simulink model "Quadcopter"  (R2019a)
settings: Solver=VariableStepAuto  StartTime=0.0  StopTime=2000  MaxStep=1e-1  RelTol=1e-3
StopFcn:
  | hold on;
  | plot3(out.out_y1.data, out.out_x1.data, out.out_z1.data, 'r');
  | plot3(out.out_y2.data, out.out_x2.data, out.out_z2.data, 'g');
  | plot3(out.out_y3.data, out.out_x3.data, out.out_z3.data, 'b');
  | plot3([0;out.out_y.data(1:1000:end)], [0;out.out_x.data(1:1000:end)], [0;out.out_z.data(1:1000:end)], '.k');
  | view(3);
  | hold off;
values from neighbouring files (symbols this model uses):
  B_phi = 1    [Control.m]
  B_psi = 1    [Control.m]
  B_theta = 1    [Control.m]
  B_z = 5    [Control.m]
  r_x12 = 8    [Control.m]
  r_x32 = 4    [Control.m]
  r_y12 = 8    [Control.m]
  r_y32 = 4    [Control.m]
undefined symbols (not defined in the file or in its folder): As, Bs, Cpsi, Cs, Cx, Cy, Cz, Ds, x01, x02, x03, y01, y02, y03, z01, z02, z03
libraries: simulink x1
(part 2 of 3)

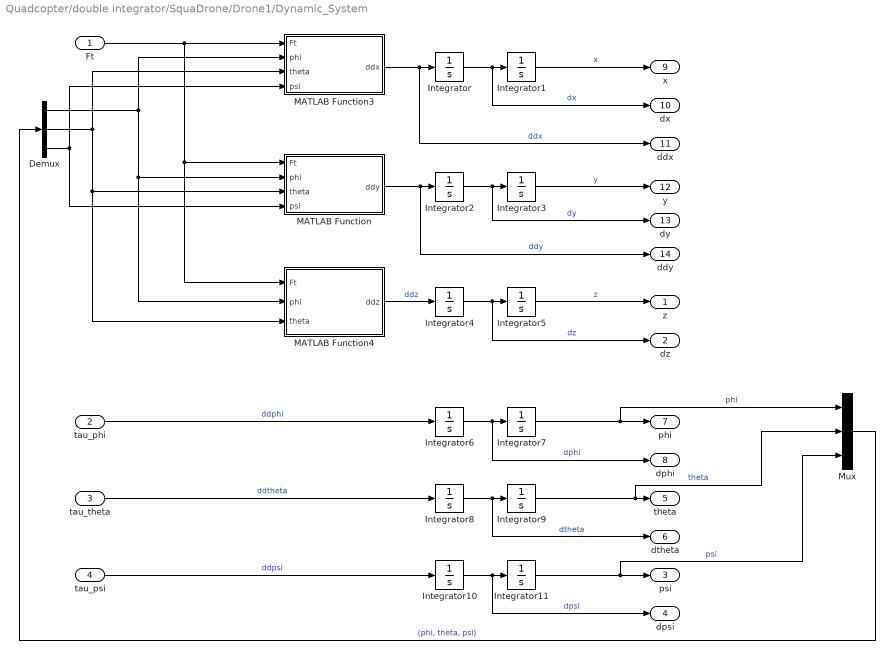
== system Quadcopter/double integrator/SquaDrone/Drone1/Dynamic_System ==
  Ft : Inport
  tau_phi : Inport  Port=2
  tau_theta : Inport  Port=3
  tau_psi : Inport  Port=4
  Demux : Demux  Outputs=3
  Integrator{,2,4,6..11} (9 alike) : Integrator
  Integrator1 : Integrator  InitialCondition=x01
  Integrator3 : Integrator  InitialCondition=y01
  Integrator5 : Integrator  InitialCondition=z01
  MATLAB Function : MATLAB Function  TreatAsAtomicUnit=on
  MATLAB Function3 : MATLAB Function  TreatAsAtomicUnit=on
  MATLAB Function4 : MATLAB Function  TreatAsAtomicUnit=on
  Mux : Mux  Inputs=3
  z : Outport
  dz : Outport  Port=2
  psi : Outport  Port=3
  dpsi : Outport  Port=4
  theta : Outport  Port=5
  dtheta : Outport  Port=6
  phi : Outport  Port=7
  dphi : Outport  Port=8
  x : Outport  Port=9
  dx : Outport  Port=10
  ddx : Outport  Port=11
  y : Outport  Port=12
  dy : Outport  Port=13
  ddy : Outport  Port=14
  wires:
  MATLAB Function3/1(ddx) -> ddx/1, Integrator/1  "ddx"
  Ft/1 -> MATLAB Function3/1(Ft), MATLAB Function4/1(Ft), MATLAB Function/1(Ft)
  Integrator/1 -> dx/1, Integrator1/1  "dx"
  Integrator1/1 -> x/1  "x"
  MATLAB Function/1(ddy) -> ddy/1, Integrator2/1  "ddy"
  Integrator2/1 -> dy/1, Integrator3/1  "dy"
  Integrator3/1 -> y/1  "y"
  MATLAB Function4/1(ddz) -> Integrator4/1  "ddz"
  Integrator4/1 -> dz/1, Integrator5/1  "dz"
  Integrator5/1 -> z/1  "z"
  tau_phi/1 -> Integrator6/1  "ddphi"
  Integrator6/1 -> dphi/1, Integrator7/1  "dphi"
  Integrator7/1 -> Mux/1, phi/1  "phi"
  Integrator9/1 -> Mux/2, theta/1  "theta"
  Integrator8/1 -> dtheta/1, Integrator9/1  "dtheta"
  tau_theta/1 -> Integrator8/1  "ddtheta"
  Integrator11/1 -> Mux/3, psi/1  "psi"
  Integrator10/1 -> dpsi/1, Integrator11/1  "dpsi"
  tau_psi/1 -> Integrator10/1  "ddpsi"
  Mux/1 -> Demux/1  "(phi, theta, psi)"
  Demux/1 -> MATLAB Function3/2(phi), MATLAB Function4/2(phi), MATLAB Function/2(phi)
  Demux/2 -> MATLAB Function3/3(theta), MATLAB Function4/3(theta), MATLAB Function/3(theta)
  Demux/3 -> MATLAB Function/4(psi), MATLAB Function3/4(psi)

== system Quadcopter/double integrator/SquaDrone/Drone2/Controller ==
  z : Inport
  dz : Inport  Port=2
  psi : Inport  Port=3
  dpsi : Inport  Port=4
  theta : Inport  Port=5
  dtheta : Inport  Port=6
  phi : Inport  Port=7
  dphi : Inport  Port=8
  zd : Inport  Port=9
  psid : Inport  Port=10
  thetad : Inport  Port=11
  dthetad : Inport  Port=12
  phid : Inport  Port=13
  dphid : Inport  Port=14
  Constant1 : Constant  Value=B_theta
  Constant14 : Constant  Value=B_z
  Constant20 : Constant  Value=B_psi
  Constant5 : Constant  Value=B_phi
  Gain{1,3,7..8} (4 alike) : Gain  Gain=2
  altitude : MATLAB Function  TreatAsAtomicUnit=on
  heading : MATLAB Function  TreatAsAtomicUnit=on
  lateral : MATLAB Function  TreatAsAtomicUnit=on
  longitudial : MATLAB Function  TreatAsAtomicUnit=on
  Ft : Outport
  tau_phi : Outport  Port=2
  tau_theta : Outport  Port=3
  tau_psi : Outport  Port=4
  wires:
  altitude/1(Ft) -> Ft/1
  longitudial/1(tau_phi) -> tau_phi/1
  lateral/1(tau_theta) -> tau_theta/1
  heading/1(tau_psi) -> tau_psi/1
  Gain7/1 -> altitude/7(M2)
  Constant14/1 -> Gain7/1, altitude/6(M1)
  Constant20/1 -> Gain8/1, heading/4(M1)
  Gain8/1 -> heading/5(M2)
  psid/1 -> heading/1(psid)
  psi/1 -> heading/2(psi)
  dpsi/1 -> heading/3(dpsi)
  theta/1 -> lateral/1(theta), altitude/4(theta)
  dtheta/1 -> lateral/2(dtheta)
  phi/1 -> longitudial/1(phi), altitude/3(phi)
  dphi/1 -> longitudial/2(dphi)
  zd/1 -> altitude/5(zd)
  z/1 -> altitude/1(z)
  dz/1 -> altitude/2(dz)
  Constant5/1 -> Gain3/1, longitudial/5(M1)
  Gain3/1 -> longitudial/6(M2)
  Constant1/1 -> Gain1/1, lateral/5(M1)
  Gain1/1 -> lateral/6(M2)
  thetad/1 -> lateral/3(thetad)
  dthetad/1 -> lateral/4(dthetad)
  phid/1 -> longitudial/3(phid)
  dphid/1 -> longitudial/4(dphid)

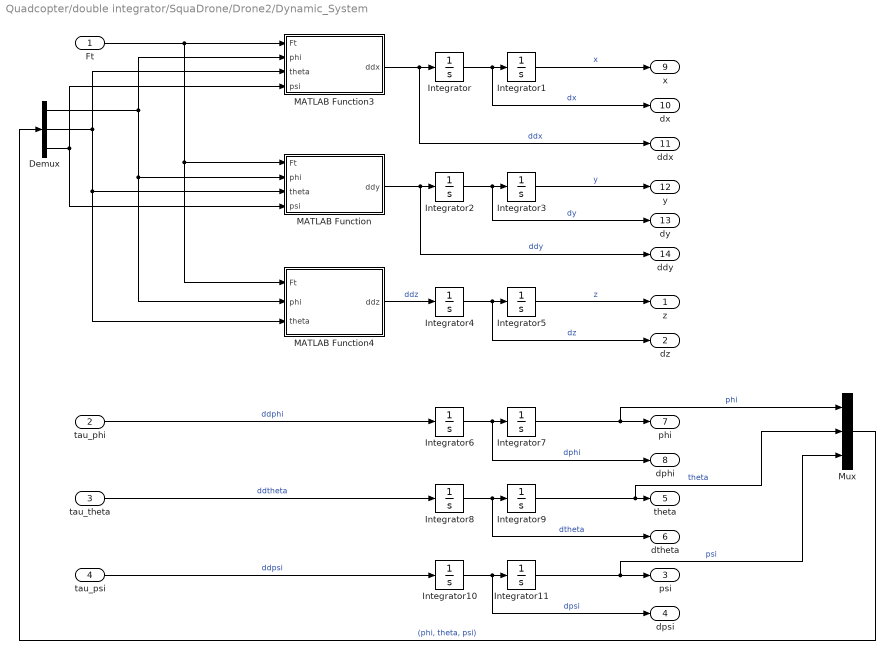
== system Quadcopter/double integrator/SquaDrone/Drone2/Dynamic_System ==
  Ft : Inport
  tau_phi : Inport  Port=2
  tau_theta : Inport  Port=3
  tau_psi : Inport  Port=4
  Demux : Demux  Outputs=3
  Integrator{,2,4,6..11} (9 alike) : Integrator
  Integrator1 : Integrator  InitialCondition=x02
  Integrator3 : Integrator  InitialCondition=y02
  Integrator5 : Integrator  InitialCondition=z02
  MATLAB Function : MATLAB Function  TreatAsAtomicUnit=on
  MATLAB Function3 : MATLAB Function  TreatAsAtomicUnit=on
  MATLAB Function4 : MATLAB Function  TreatAsAtomicUnit=on
  Mux : Mux  Inputs=3
  z : Outport
  dz : Outport  Port=2
  psi : Outport  Port=3
  dpsi : Outport  Port=4
  theta : Outport  Port=5
  dtheta : Outport  Port=6
  phi : Outport  Port=7
  dphi : Outport  Port=8
  x : Outport  Port=9
  dx : Outport  Port=10
  ddx : Outport  Port=11
  y : Outport  Port=12
  dy : Outport  Port=13
  ddy : Outport  Port=14
  wires:
  MATLAB Function3/1(ddx) -> ddx/1, Integrator/1  "ddx"
  Ft/1 -> MATLAB Function3/1(Ft), MATLAB Function4/1(Ft), MATLAB Function/1(Ft)
  Integrator/1 -> dx/1, Integrator1/1  "dx"
  Integrator1/1 -> x/1  "x"
  MATLAB Function/1(ddy) -> ddy/1, Integrator2/1  "ddy"
  Integrator2/1 -> dy/1, Integrator3/1  "dy"
  Integrator3/1 -> y/1  "y"
  MATLAB Function4/1(ddz) -> Integrator4/1  "ddz"
  Integrator4/1 -> dz/1, Integrator5/1  "dz"
  Integrator5/1 -> z/1  "z"
  tau_phi/1 -> Integrator6/1  "ddphi"
  Integrator6/1 -> dphi/1, Integrator7/1  "dphi"
  Integrator7/1 -> Mux/1, phi/1  "phi"
  Integrator9/1 -> Mux/2, theta/1  "theta"
  Integrator8/1 -> dtheta/1, Integrator9/1  "dtheta"
  tau_theta/1 -> Integrator8/1  "ddtheta"
  Integrator11/1 -> Mux/3, psi/1  "psi"
  Integrator10/1 -> dpsi/1, Integrator11/1  "dpsi"
  tau_psi/1 -> Integrator10/1  "ddpsi"
  Mux/1 -> Demux/1  "(phi, theta, psi)"
  Demux/1 -> MATLAB Function3/2(phi), MATLAB Function4/2(phi), MATLAB Function/2(phi)
  Demux/2 -> MATLAB Function3/3(theta), MATLAB Function4/3(theta), MATLAB Function/3(theta)
  Demux/3 -> MATLAB Function/4(psi), MATLAB Function3/4(psi)

== system Quadcopter/double integrator/SquaDrone/Drone3/Controller ==
  z : Inport
  dz : Inport  Port=2
  psi : Inport  Port=3
  dpsi : Inport  Port=4
  theta : Inport  Port=5
  dtheta : Inport  Port=6
  phi : Inport  Port=7
  dphi : Inport  Port=8
  zd : Inport  Port=9
  psid : Inport  Port=10
  thetad : Inport  Port=11
  dthetad : Inport  Port=12
  phid : Inport  Port=13
  dphid : Inport  Port=14
  Constant1 : Constant  Value=B_theta
  Constant14 : Constant  Value=B_z
  Constant20 : Constant  Value=B_psi
  Constant5 : Constant  Value=B_phi
  Gain{1,3,7..8} (4 alike) : Gain  Gain=2
  altitude : MATLAB Function  TreatAsAtomicUnit=on
  heading : MATLAB Function  TreatAsAtomicUnit=on
  lateral : MATLAB Function  TreatAsAtomicUnit=on
  longitudial : MATLAB Function  TreatAsAtomicUnit=on
  Ft : Outport
  tau_phi : Outport  Port=2
  tau_theta : Outport  Port=3
  tau_psi : Outport  Port=4
  wires:
  altitude/1(Ft) -> Ft/1
  longitudial/1(tau_phi) -> tau_phi/1
  lateral/1(tau_theta) -> tau_theta/1
  heading/1(tau_psi) -> tau_psi/1
  Gain7/1 -> altitude/7(M2)
  Constant14/1 -> Gain7/1, altitude/6(M1)
  Constant20/1 -> Gain8/1, heading/4(M1)
  Gain8/1 -> heading/5(M2)
  psid/1 -> heading/1(psid)
  psi/1 -> heading/2(psi)
  dpsi/1 -> heading/3(dpsi)
  theta/1 -> lateral/1(theta), altitude/4(theta)
  dtheta/1 -> lateral/2(dtheta)
  phi/1 -> longitudial/1(phi), altitude/3(phi)
  dphi/1 -> longitudial/2(dphi)
  zd/1 -> altitude/5(zd)
  z/1 -> altitude/1(z)
  dz/1 -> altitude/2(dz)
  Constant5/1 -> Gain3/1, longitudial/5(M1)
  Gain3/1 -> longitudial/6(M2)
  Constant1/1 -> Gain1/1, lateral/5(M1)
  Gain1/1 -> lateral/6(M2)
  thetad/1 -> lateral/3(thetad)
  dthetad/1 -> lateral/4(dthetad)
  phid/1 -> longitudial/3(phid)
  dphid/1 -> longitudial/4(dphid)

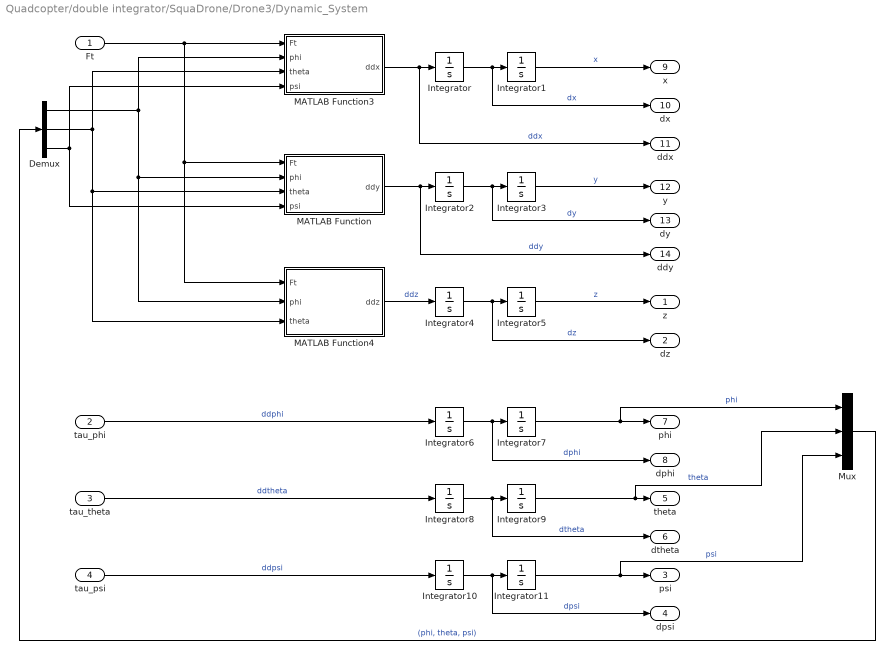
== system Quadcopter/double integrator/SquaDrone/Drone3/Dynamic_System ==
  Ft : Inport
  tau_phi : Inport  Port=2
  tau_theta : Inport  Port=3
  tau_psi : Inport  Port=4
  Demux : Demux  Outputs=3
  Integrator{,2,4,6..11} (9 alike) : Integrator
  Integrator1 : Integrator  InitialCondition=x03
  Integrator3 : Integrator  InitialCondition=y03
  Integrator5 : Integrator  InitialCondition=z03
  MATLAB Function : MATLAB Function  TreatAsAtomicUnit=on
  MATLAB Function3 : MATLAB Function  TreatAsAtomicUnit=on
  MATLAB Function4 : MATLAB Function  TreatAsAtomicUnit=on
  Mux : Mux  Inputs=3
  z : Outport
  dz : Outport  Port=2
  psi : Outport  Port=3
  dpsi : Outport  Port=4
  theta : Outport  Port=5
  dtheta : Outport  Port=6
  phi : Outport  Port=7
  dphi : Outport  Port=8
  x : Outport  Port=9
  dx : Outport  Port=10
  ddx : Outport  Port=11
  y : Outport  Port=12
  dy : Outport  Port=13
  ddy : Outport  Port=14
  wires:
  MATLAB Function3/1(ddx) -> ddx/1, Integrator/1  "ddx"
  Ft/1 -> MATLAB Function3/1(Ft), MATLAB Function4/1(Ft), MATLAB Function/1(Ft)
  Integrator/1 -> dx/1, Integrator1/1  "dx"
  Integrator1/1 -> x/1  "x"
  MATLAB Function/1(ddy) -> ddy/1, Integrator2/1  "ddy"
  Integrator2/1 -> dy/1, Integrator3/1  "dy"
  Integrator3/1 -> y/1  "y"
  MATLAB Function4/1(ddz) -> Integrator4/1  "ddz"
  Integrator4/1 -> dz/1, Integrator5/1  "dz"
  Integrator5/1 -> z/1  "z"
  tau_phi/1 -> Integrator6/1  "ddphi"
  Integrator6/1 -> dphi/1, Integrator7/1  "dphi"
  Integrator7/1 -> Mux/1, phi/1  "phi"
  Integrator9/1 -> Mux/2, theta/1  "theta"
  Integrator8/1 -> dtheta/1, Integrator9/1  "dtheta"
  tau_theta/1 -> Integrator8/1  "ddtheta"
  Integrator11/1 -> Mux/3, psi/1  "psi"
  Integrator10/1 -> dpsi/1, Integrator11/1  "dpsi"
  tau_psi/1 -> Integrator10/1  "ddpsi"
  Mux/1 -> Demux/1  "(phi, theta, psi)"
  Demux/1 -> MATLAB Function3/2(phi), MATLAB Function4/2(phi), MATLAB Function/2(phi)
  Demux/2 -> MATLAB Function3/3(theta), MATLAB Function4/3(theta), MATLAB Function/3(theta)
  Demux/3 -> MATLAB Function/4(psi), MATLAB Function3/4(psi)

== system Quadcopter/scheme - double integrator/SquaDrone/Drone1/Controller ==
  z : Inport
  dz : Inport  Port=2
  psi : Inport  Port=3
  dpsi : Inport  Port=4
  theta : Inport  Port=5
  dtheta : Inport  Port=6
  phi : Inport  Port=7
  dphi : Inport  Port=8
  zd : Inport  Port=9
  psid : Inport  Port=10
  thetad : Inport  Port=11
  dthetad : Inport  Port=12
  phid : Inport  Port=13
  dphid : Inport  Port=14
  Constant1 : Constant  Value=B_theta
  Constant14 : Constant  Value=B_z
  Constant20 : Constant  Value=B_psi
  Constant5 : Constant  Value=B_phi
  Gain{1,3,7..8} (4 alike) : Gain  Gain=2
  altitude : MATLAB Function  TreatAsAtomicUnit=on
  heading : MATLAB Function  TreatAsAtomicUnit=on
  lateral : MATLAB Function  TreatAsAtomicUnit=on
  longitudial : MATLAB Function  TreatAsAtomicUnit=on
  Ft : Outport
  tau_phi : Outport  Port=2
  tau_theta : Outport  Port=3
  tau_psi : Outport  Port=4
  wires:
  altitude/1(Ft) -> Ft/1
  longitudial/1(tau_phi) -> tau_phi/1
  lateral/1(tau_theta) -> tau_theta/1
  heading/1(tau_psi) -> tau_psi/1
  Gain7/1 -> altitude/7(M2)
  Constant14/1 -> Gain7/1, altitude/6(M1)
  Constant20/1 -> Gain8/1, heading/4(M1)
  Gain8/1 -> heading/5(M2)
  psid/1 -> heading/1(psid)
  psi/1 -> heading/2(psi)
  dpsi/1 -> heading/3(dpsi)
  theta/1 -> lateral/1(theta), altitude/4(theta)
  dtheta/1 -> lateral/2(dtheta)
  phi/1 -> longitudial/1(phi), altitude/3(phi)
  dphi/1 -> longitudial/2(dphi)
  zd/1 -> altitude/5(zd)
  z/1 -> altitude/1(z)
  dz/1 -> altitude/2(dz)
  Constant5/1 -> Gain3/1, longitudial/5(M1)
  Gain3/1 -> longitudial/6(M2)
  Constant1/1 -> Gain1/1, lateral/5(M1)
  Gain1/1 -> lateral/6(M2)
  thetad/1 -> lateral/3(thetad)
  dthetad/1 -> lateral/4(dthetad)
  phid/1 -> longitudial/3(phid)
  dphid/1 -> longitudial/4(dphid)

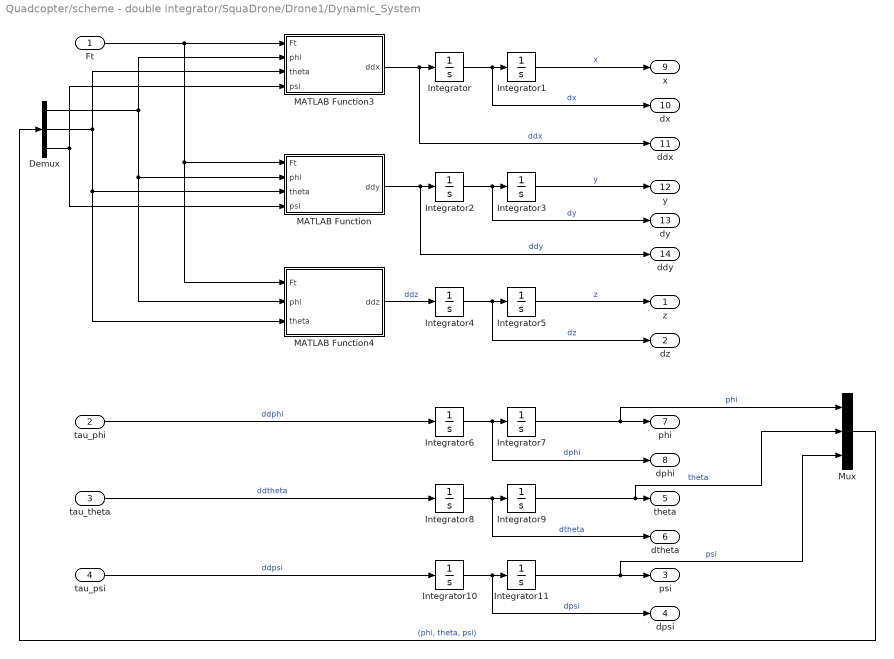
== system Quadcopter/scheme - double integrator/SquaDrone/Drone1/Dynamic_System ==
  Ft : Inport
  tau_phi : Inport  Port=2
  tau_theta : Inport  Port=3
  tau_psi : Inport  Port=4
  Demux : Demux  Outputs=3
  Integrator{,2,4,6..11} (9 alike) : Integrator
  Integrator1 : Integrator  InitialCondition=x01
  Integrator3 : Integrator  InitialCondition=y01
  Integrator5 : Integrator  InitialCondition=z01
  MATLAB Function : MATLAB Function  TreatAsAtomicUnit=on
  MATLAB Function3 : MATLAB Function  TreatAsAtomicUnit=on
  MATLAB Function4 : MATLAB Function  TreatAsAtomicUnit=on
  Mux : Mux  Inputs=3
  z : Outport
  dz : Outport  Port=2
  psi : Outport  Port=3
  dpsi : Outport  Port=4
  theta : Outport  Port=5
  dtheta : Outport  Port=6
  phi : Outport  Port=7
  dphi : Outport  Port=8
  x : Outport  Port=9
  dx : Outport  Port=10
  ddx : Outport  Port=11
  y : Outport  Port=12
  dy : Outport  Port=13
  ddy : Outport  Port=14
  wires:
  MATLAB Function3/1(ddx) -> ddx/1, Integrator/1  "ddx"
  Ft/1 -> MATLAB Function3/1(Ft), MATLAB Function4/1(Ft), MATLAB Function/1(Ft)
  Integrator/1 -> dx/1, Integrator1/1  "dx"
  Integrator1/1 -> x/1  "x"
  MATLAB Function/1(ddy) -> ddy/1, Integrator2/1  "ddy"
  Integrator2/1 -> dy/1, Integrator3/1  "dy"
  Integrator3/1 -> y/1  "y"
  MATLAB Function4/1(ddz) -> Integrator4/1  "ddz"
  Integrator4/1 -> dz/1, Integrator5/1  "dz"
  Integrator5/1 -> z/1  "z"
  tau_phi/1 -> Integrator6/1  "ddphi"
  Integrator6/1 -> dphi/1, Integrator7/1  "dphi"
  Integrator7/1 -> Mux/1, phi/1  "phi"
  Integrator9/1 -> Mux/2, theta/1  "theta"
  Integrator8/1 -> dtheta/1, Integrator9/1  "dtheta"
  tau_theta/1 -> Integrator8/1  "ddtheta"
  Integrator11/1 -> Mux/3, psi/1  "psi"
  Integrator10/1 -> dpsi/1, Integrator11/1  "dpsi"
  tau_psi/1 -> Integrator10/1  "ddpsi"
  Mux/1 -> Demux/1  "(phi, theta, psi)"
  Demux/1 -> MATLAB Function3/2(phi), MATLAB Function4/2(phi), MATLAB Function/2(phi)
  Demux/2 -> MATLAB Function3/3(theta), MATLAB Function4/3(theta), MATLAB Function/3(theta)
  Demux/3 -> MATLAB Function/4(psi), MATLAB Function3/4(psi)

== system Quadcopter/scheme - double integrator/SquaDrone/Drone2/Controller ==
  z : Inport
  dz : Inport  Port=2
  psi : Inport  Port=3
  dpsi : Inport  Port=4
  theta : Inport  Port=5
  dtheta : Inport  Port=6
  phi : Inport  Port=7
  dphi : Inport  Port=8
  zd : Inport  Port=9
  psid : Inport  Port=10
  thetad : Inport  Port=11
  dthetad : Inport  Port=12
  phid : Inport  Port=13
  dphid : Inport  Port=14
  Constant1 : Constant  Value=B_theta
  Constant14 : Constant  Value=B_z
  Constant20 : Constant  Value=B_psi
  Constant5 : Constant  Value=B_phi
  Gain{1,3,7..8} (4 alike) : Gain  Gain=2
  altitude : MATLAB Function  TreatAsAtomicUnit=on
  heading : MATLAB Function  TreatAsAtomicUnit=on
  lateral : MATLAB Function  TreatAsAtomicUnit=on
  longitudial : MATLAB Function  TreatAsAtomicUnit=on
  Ft : Outport
  tau_phi : Outport  Port=2
  tau_theta : Outport  Port=3
  tau_psi : Outport  Port=4
  wires:
  altitude/1(Ft) -> Ft/1
  longitudial/1(tau_phi) -> tau_phi/1
  lateral/1(tau_theta) -> tau_theta/1
  heading/1(tau_psi) -> tau_psi/1
  Gain7/1 -> altitude/7(M2)
  Constant14/1 -> Gain7/1, altitude/6(M1)
  Constant20/1 -> Gain8/1, heading/4(M1)
  Gain8/1 -> heading/5(M2)
  psid/1 -> heading/1(psid)
  psi/1 -> heading/2(psi)
  dpsi/1 -> heading/3(dpsi)
  theta/1 -> lateral/1(theta), altitude/4(theta)
  dtheta/1 -> lateral/2(dtheta)
  phi/1 -> longitudial/1(phi), altitude/3(phi)
  dphi/1 -> longitudial/2(dphi)
  zd/1 -> altitude/5(zd)
  z/1 -> altitude/1(z)
  dz/1 -> altitude/2(dz)
  Constant5/1 -> Gain3/1, longitudial/5(M1)
  Gain3/1 -> longitudial/6(M2)
  Constant1/1 -> Gain1/1, lateral/5(M1)
  Gain1/1 -> lateral/6(M2)
  thetad/1 -> lateral/3(thetad)
  dthetad/1 -> lateral/4(dthetad)
  phid/1 -> longitudial/3(phid)
  dphid/1 -> longitudial/4(dphid)

== system Quadcopter/scheme - double integrator/SquaDrone/Drone2/Dynamic_System ==
  Ft : Inport
  tau_phi : Inport  Port=2
  tau_theta : Inport  Port=3
  tau_psi : Inport  Port=4
  Demux : Demux  Outputs=3
  Integrator{,2,4,6..11} (9 alike) : Integrator
  Integrator1 : Integrator  InitialCondition=x01
  Integrator3 : Integrator  InitialCondition=y01
  Integrator5 : Integrator  InitialCondition=z01
  MATLAB Function : MATLAB Function  TreatAsAtomicUnit=on
  MATLAB Function3 : MATLAB Function  TreatAsAtomicUnit=on
  MATLAB Function4 : MATLAB Function  TreatAsAtomicUnit=on
  Mux : Mux  Inputs=3
  z : Outport
  dz : Outport  Port=2
  psi : Outport  Port=3
  dpsi : Outport  Port=4
  theta : Outport  Port=5
  dtheta : Outport  Port=6
  phi : Outport  Port=7
  dphi : Outport  Port=8
  x : Outport  Port=9
  dx : Outport  Port=10
  ddx : Outport  Port=11
  y : Outport  Port=12
  dy : Outport  Port=13
  ddy : Outport  Port=14
  wires:
  MATLAB Function3/1(ddx) -> ddx/1, Integrator/1  "ddx"
  Ft/1 -> MATLAB Function3/1(Ft), MATLAB Function4/1(Ft), MATLAB Function/1(Ft)
  Integrator/1 -> dx/1, Integrator1/1  "dx"
  Integrator1/1 -> x/1  "x"
  MATLAB Function/1(ddy) -> ddy/1, Integrator2/1  "ddy"
  Integrator2/1 -> dy/1, Integrator3/1  "dy"
  Integrator3/1 -> y/1  "y"
  MATLAB Function4/1(ddz) -> Integrator4/1  "ddz"
  Integrator4/1 -> dz/1, Integrator5/1  "dz"
  Integrator5/1 -> z/1  "z"
  tau_phi/1 -> Integrator6/1  "ddphi"
  Integrator6/1 -> dphi/1, Integrator7/1  "dphi"
  Integrator7/1 -> Mux/1, phi/1  "phi"
  Integrator9/1 -> Mux/2, theta/1  "theta"
  Integrator8/1 -> dtheta/1, Integrator9/1  "dtheta"
  tau_theta/1 -> Integrator8/1  "ddtheta"
  Integrator11/1 -> Mux/3, psi/1  "psi"
  Integrator10/1 -> dpsi/1, Integrator11/1  "dpsi"
  tau_psi/1 -> Integrator10/1  "ddpsi"
  Mux/1 -> Demux/1  "(phi, theta, psi)"
  Demux/1 -> MATLAB Function3/2(phi), MATLAB Function4/2(phi), MATLAB Function/2(phi)
  Demux/2 -> MATLAB Function3/3(theta), MATLAB Function4/3(theta), MATLAB Function/3(theta)
  Demux/3 -> MATLAB Function/4(psi), MATLAB Function3/4(psi)

== system Quadcopter/scheme - double integrator/SquaDrone/Drone3/Controller ==
  z : Inport
  dz : Inport  Port=2
  psi : Inport  Port=3
  dpsi : Inport  Port=4
  theta : Inport  Port=5
  dtheta : Inport  Port=6
  phi : Inport  Port=7
  dphi : Inport  Port=8
  zd : Inport  Port=9
  psid : Inport  Port=10
  thetad : Inport  Port=11
  dthetad : Inport  Port=12
  phid : Inport  Port=13
  dphid : Inport  Port=14
  Constant1 : Constant  Value=B_theta
  Constant14 : Constant  Value=B_z
  Constant20 : Constant  Value=B_psi
  Constant5 : Constant  Value=B_phi
  Gain{1,3,7..8} (4 alike) : Gain  Gain=2
  altitude : MATLAB Function  TreatAsAtomicUnit=on
  heading : MATLAB Function  TreatAsAtomicUnit=on
  lateral : MATLAB Function  TreatAsAtomicUnit=on
  longitudial : MATLAB Function  TreatAsAtomicUnit=on
  Ft : Outport
  tau_phi : Outport  Port=2
  tau_theta : Outport  Port=3
  tau_psi : Outport  Port=4
  wires:
  altitude/1(Ft) -> Ft/1
  longitudial/1(tau_phi) -> tau_phi/1
  lateral/1(tau_theta) -> tau_theta/1
  heading/1(tau_psi) -> tau_psi/1
  Gain7/1 -> altitude/7(M2)
  Constant14/1 -> Gain7/1, altitude/6(M1)
  Constant20/1 -> Gain8/1, heading/4(M1)
  Gain8/1 -> heading/5(M2)
  psid/1 -> heading/1(psid)
  psi/1 -> heading/2(psi)
  dpsi/1 -> heading/3(dpsi)
  theta/1 -> lateral/1(theta), altitude/4(theta)
  dtheta/1 -> lateral/2(dtheta)
  phi/1 -> longitudial/1(phi), altitude/3(phi)
  dphi/1 -> longitudial/2(dphi)
  zd/1 -> altitude/5(zd)
  z/1 -> altitude/1(z)
  dz/1 -> altitude/2(dz)
  Constant5/1 -> Gain3/1, longitudial/5(M1)
  Gain3/1 -> longitudial/6(M2)
  Constant1/1 -> Gain1/1, lateral/5(M1)
  Gain1/1 -> lateral/6(M2)
  thetad/1 -> lateral/3(thetad)
  dthetad/1 -> lateral/4(dthetad)
  phid/1 -> longitudial/3(phid)
  dphid/1 -> longitudial/4(dphid)

== system Quadcopter/scheme - double integrator/SquaDrone/Drone3/Dynamic_System ==
  Ft : Inport
  tau_phi : Inport  Port=2
  tau_theta : Inport  Port=3
  tau_psi : Inport  Port=4
  Demux : Demux  Outputs=3
  Integrator{,2,4,6..11} (9 alike) : Integrator
  Integrator1 : Integrator  InitialCondition=x01
  Integrator3 : Integrator  InitialCondition=y01
  Integrator5 : Integrator  InitialCondition=z01
  MATLAB Function : MATLAB Function  TreatAsAtomicUnit=on
  MATLAB Function3 : MATLAB Function  TreatAsAtomicUnit=on
  MATLAB Function4 : MATLAB Function  TreatAsAtomicUnit=on
  Mux : Mux  Inputs=3
  z : Outport
  dz : Outport  Port=2
  psi : Outport  Port=3
  dpsi : Outport  Port=4
  theta : Outport  Port=5
  dtheta : Outport  Port=6
  phi : Outport  Port=7
  dphi : Outport  Port=8
  x : Outport  Port=9
  dx : Outport  Port=10
  ddx : Outport  Port=11
  y : Outport  Port=12
  dy : Outport  Port=13
  ddy : Outport  Port=14
  wires:
  MATLAB Function3/1(ddx) -> ddx/1, Integrator/1  "ddx"
  Ft/1 -> MATLAB Function3/1(Ft), MATLAB Function4/1(Ft), MATLAB Function/1(Ft)
  Integrator/1 -> dx/1, Integrator1/1  "dx"
  Integrator1/1 -> x/1  "x"
  MATLAB Function/1(ddy) -> ddy/1, Integrator2/1  "ddy"
  Integrator2/1 -> dy/1, Integrator3/1  "dy"
  Integrator3/1 -> y/1  "y"
  MATLAB Function4/1(ddz) -> Integrator4/1  "ddz"
  Integrator4/1 -> dz/1, Integrator5/1  "dz"
  Integrator5/1 -> z/1  "z"
  tau_phi/1 -> Integrator6/1  "ddphi"
  Integrator6/1 -> dphi/1, Integrator7/1  "dphi"
  Integrator7/1 -> Mux/1, phi/1  "phi"
  Integrator9/1 -> Mux/2, theta/1  "theta"
  Integrator8/1 -> dtheta/1, Integrator9/1  "dtheta"
  tau_theta/1 -> Integrator8/1  "ddtheta"
  Integrator11/1 -> Mux/3, psi/1  "psi"
  Integrator10/1 -> dpsi/1, Integrator11/1  "dpsi"
  tau_psi/1 -> Integrator10/1  "ddpsi"
  Mux/1 -> Demux/1  "(phi, theta, psi)"
  Demux/1 -> MATLAB Function3/2(phi), MATLAB Function4/2(phi), MATLAB Function/2(phi)
  Demux/2 -> MATLAB Function3/3(theta), MATLAB Function4/3(theta), MATLAB Function/3(theta)
  Demux/3 -> MATLAB Function/4(psi), MATLAB Function3/4(psi)

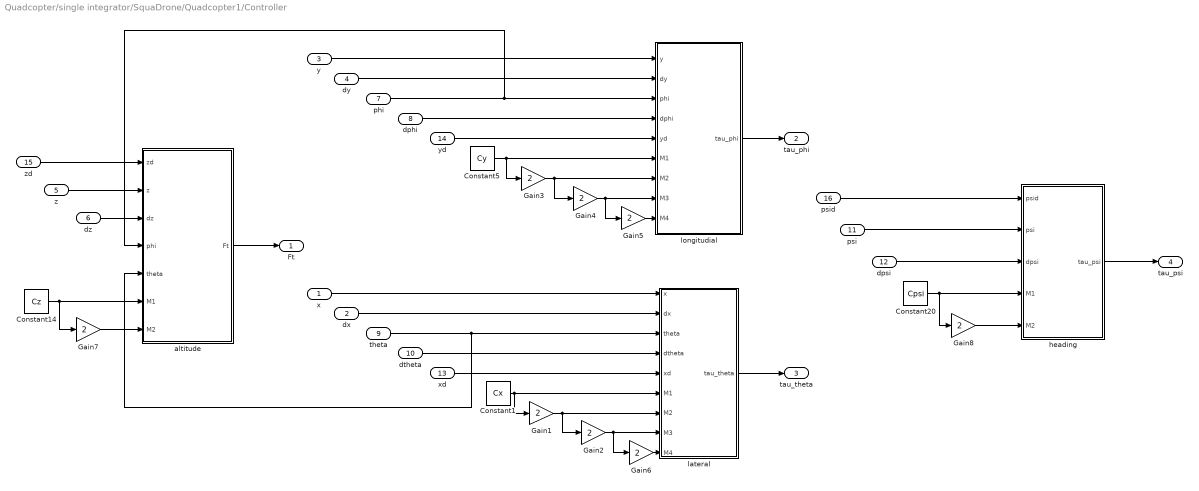
== system Quadcopter/single integrator/SquaDrone/Quadcopter1/Controller ==
  x : Inport
  dx : Inport  Port=2
  y : Inport  Port=3
  dy : Inport  Port=4
  z : Inport  Port=5
  dz : Inport  Port=6
  phi : Inport  Port=7
  dphi : Inport  Port=8
  theta : Inport  Port=9
  dtheta : Inport  Port=10
  psi : Inport  Port=11
  dpsi : Inport  Port=12
  xd : Inport  Port=13
  yd : Inport  Port=14
  zd : Inport  Port=15
  psid : Inport  Port=16
  Constant1 : Constant  Value=Cx
  Constant14 : Constant  Value=Cz
  Constant20 : Constant  Value=Cpsi
  Constant5 : Constant  Value=Cy
  Gain{1..8} (8 alike) : Gain  Gain=2
  altitude : MATLAB Function  TreatAsAtomicUnit=on
  heading : MATLAB Function  TreatAsAtomicUnit=on
  lateral : MATLAB Function  TreatAsAtomicUnit=on
  longitudial : MATLAB Function  TreatAsAtomicUnit=on
  Ft : Outport
  tau_phi : Outport  Port=2
  tau_theta : Outport  Port=3
  tau_psi : Outport  Port=4
  wires:
  altitude/1(Ft) -> Ft/1
  longitudial/1(tau_phi) -> tau_phi/1
  lateral/1(tau_theta) -> tau_theta/1
  heading/1(tau_psi) -> tau_psi/1
  Gain7/1 -> altitude/7(M2)
  Constant14/1 -> Gain7/1, altitude/6(M1)
  Constant20/1 -> Gain8/1, heading/4(M1)
  Gain8/1 -> heading/5(M2)
  psid/1 -> heading/1(psid)
  psi/1 -> heading/2(psi)
  dpsi/1 -> heading/3(dpsi)
  dx/1 -> lateral/2(dx)
  x/1 -> lateral/1(x)
  theta/1 -> lateral/3(theta), altitude/5(theta)
  dtheta/1 -> lateral/4(dtheta)
  y/1 -> longitudial/1(y)
  dy/1 -> longitudial/2(dy)
  phi/1 -> altitude/4(phi), longitudial/3(phi)
  dphi/1 -> longitudial/4(dphi)
  xd/1 -> lateral/5(xd)
  yd/1 -> longitudial/5(yd)
  zd/1 -> altitude/1(zd)
  z/1 -> altitude/2(z)
  dz/1 -> altitude/3(dz)
  Gain4/1 -> longitudial/8(M3), Gain5/1
  Constant5/1 -> longitudial/6(M1), Gain3/1
  Gain3/1 -> longitudial/7(M2), Gain4/1
  Gain5/1 -> longitudial/9(M4)
  Gain2/1 -> lateral/8(M3), Gain6/1
  Constant1/1 -> lateral/6(M1), Gain1/1
  Gain1/1 -> lateral/7(M2), Gain2/1
  Gain6/1 -> lateral/9(M4)

== system Quadcopter/single integrator/SquaDrone/Quadcopter1/Dynamic_System ==
  Ft : Inport
  tau_phi : Inport  Port=2
  tau_theta : Inport  Port=3
  tau_psi : Inport  Port=4
  Demux : Demux  Outputs=3
  Integrator{,1..11} (12 alike) : Integrator
  MATLAB Function : MATLAB Function  TreatAsAtomicUnit=on
  MATLAB Function3 : MATLAB Function  TreatAsAtomicUnit=on
  MATLAB Function4 : MATLAB Function  TreatAsAtomicUnit=on
  Mux : Mux  Inputs=3
  x : Outport
  dx : Outport  Port=2
  y : Outport  Port=3
  dy : Outport  Port=4
  z : Outport  Port=5
  dz : Outport  Port=6
  phi : Outport  Port=7
  dphi : Outport  Port=8
  theta : Outport  Port=9
  dtheta : Outport  Port=10
  psi : Outport  Port=11
  dpsi : Outport  Port=12
  wires:
  MATLAB Function3/1(ddx) -> Integrator/1  "ddx"
  Ft/1 -> MATLAB Function3/1(Ft), MATLAB Function4/1(Ft), MATLAB Function/1(Ft)
  Integrator/1 -> dx/1, Integrator1/1  "dx"
  Integrator1/1 -> x/1  "x"
  MATLAB Function/1(ddy) -> Integrator2/1  "ddy"
  Integrator2/1 -> dy/1, Integrator3/1  "dy"
  Integrator3/1 -> y/1  "y"
  MATLAB Function4/1(ddz) -> Integrator4/1  "ddz"
  Integrator4/1 -> dz/1, Integrator5/1  "dz"
  Integrator5/1 -> z/1  "z"
  tau_phi/1 -> Integrator6/1  "ddphi"
  Integrator6/1 -> dphi/1, Integrator7/1  "dphi"
  Integrator7/1 -> Mux/1, phi/1  "phi"
  Integrator9/1 -> Mux/2, theta/1  "theta"
  Integrator8/1 -> dtheta/1, Integrator9/1  "dtheta"
  tau_theta/1 -> Integrator8/1  "ddtheta"
  Integrator11/1 -> Mux/3, psi/1  "psi"
  Integrator10/1 -> dpsi/1, Integrator11/1  "dpsi"
  tau_psi/1 -> Integrator10/1  "ddpsi"
  Mux/1 -> Demux/1  "(phi, theta, psi)"
  Demux/1 -> MATLAB Function3/2(phi), MATLAB Function4/2(phi), MATLAB Function/2(phi)
  Demux/2 -> MATLAB Function3/3(theta), MATLAB Function4/3(theta), MATLAB Function/3(theta)
  Demux/3 -> MATLAB Function/4(psi), MATLAB Function3/4(psi)

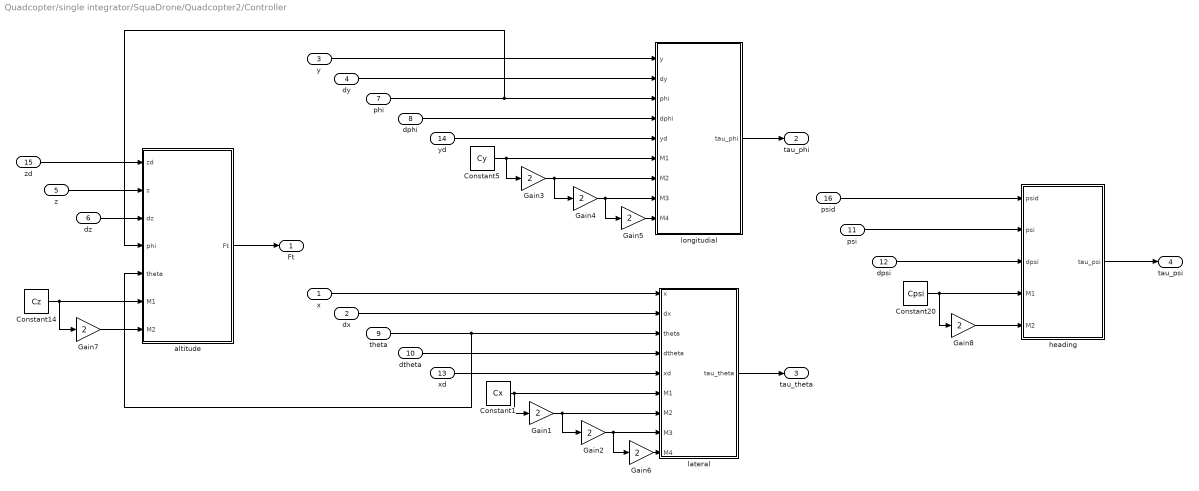
== system Quadcopter/single integrator/SquaDrone/Quadcopter2/Controller ==
  x : Inport
  dx : Inport  Port=2
  y : Inport  Port=3
  dy : Inport  Port=4
  z : Inport  Port=5
  dz : Inport  Port=6
  phi : Inport  Port=7
  dphi : Inport  Port=8
  theta : Inport  Port=9
  dtheta : Inport  Port=10
  psi : Inport  Port=11
  dpsi : Inport  Port=12
  xd : Inport  Port=13
  yd : Inport  Port=14
  zd : Inport  Port=15
  psid : Inport  Port=16
  Constant1 : Constant  Value=Cx
  Constant14 : Constant  Value=Cz
  Constant20 : Constant  Value=Cpsi
  Constant5 : Constant  Value=Cy
  Gain{1..8} (8 alike) : Gain  Gain=2
  altitude : MATLAB Function  TreatAsAtomicUnit=on
  heading : MATLAB Function  TreatAsAtomicUnit=on
  lateral : MATLAB Function  TreatAsAtomicUnit=on
  longitudial : MATLAB Function  TreatAsAtomicUnit=on
  Ft : Outport
  tau_phi : Outport  Port=2
  tau_theta : Outport  Port=3
  tau_psi : Outport  Port=4
  wires:
  altitude/1(Ft) -> Ft/1
  longitudial/1(tau_phi) -> tau_phi/1
  lateral/1(tau_theta) -> tau_theta/1
  heading/1(tau_psi) -> tau_psi/1
  Gain7/1 -> altitude/7(M2)
  Constant14/1 -> Gain7/1, altitude/6(M1)
  Constant20/1 -> Gain8/1, heading/4(M1)
  Gain8/1 -> heading/5(M2)
  psid/1 -> heading/1(psid)
  psi/1 -> heading/2(psi)
  dpsi/1 -> heading/3(dpsi)
  dx/1 -> lateral/2(dx)
  x/1 -> lateral/1(x)
  theta/1 -> lateral/3(theta), altitude/5(theta)
  dtheta/1 -> lateral/4(dtheta)
  y/1 -> longitudial/1(y)
  dy/1 -> longitudial/2(dy)
  phi/1 -> altitude/4(phi), longitudial/3(phi)
  dphi/1 -> longitudial/4(dphi)
  xd/1 -> lateral/5(xd)
  yd/1 -> longitudial/5(yd)
  zd/1 -> altitude/1(zd)
  z/1 -> altitude/2(z)
  dz/1 -> altitude/3(dz)
  Gain4/1 -> longitudial/8(M3), Gain5/1
  Constant5/1 -> longitudial/6(M1), Gain3/1
  Gain3/1 -> longitudial/7(M2), Gain4/1
  Gain5/1 -> longitudial/9(M4)
  Gain2/1 -> lateral/8(M3), Gain6/1
  Constant1/1 -> lateral/6(M1), Gain1/1
  Gain1/1 -> lateral/7(M2), Gain2/1
  Gain6/1 -> lateral/9(M4)

== system Quadcopter/single integrator/SquaDrone/Quadcopter2/Dynamic_System ==
  Ft : Inport
  tau_phi : Inport  Port=2
  tau_theta : Inport  Port=3
  tau_psi : Inport  Port=4
  Demux : Demux  Outputs=3
  Integrator{,1..11} (12 alike) : Integrator
  MATLAB Function : MATLAB Function  TreatAsAtomicUnit=on
  MATLAB Function3 : MATLAB Function  TreatAsAtomicUnit=on
  MATLAB Function4 : MATLAB Function  TreatAsAtomicUnit=on
  Mux : Mux  Inputs=3
  x : Outport
  dx : Outport  Port=2
  y : Outport  Port=3
  dy : Outport  Port=4
  z : Outport  Port=5
  dz : Outport  Port=6
  phi : Outport  Port=7
  dphi : Outport  Port=8
  theta : Outport  Port=9
  dtheta : Outport  Port=10
  psi : Outport  Port=11
  dpsi : Outport  Port=12
  wires:
  MATLAB Function3/1(ddx) -> Integrator/1  "ddx"
  Ft/1 -> MATLAB Function3/1(Ft), MATLAB Function4/1(Ft), MATLAB Function/1(Ft)
  Integrator/1 -> dx/1, Integrator1/1  "dx"
  Integrator1/1 -> x/1  "x"
  MATLAB Function/1(ddy) -> Integrator2/1  "ddy"
  Integrator2/1 -> dy/1, Integrator3/1  "dy"
  Integrator3/1 -> y/1  "y"
  MATLAB Function4/1(ddz) -> Integrator4/1  "ddz"
  Integrator4/1 -> dz/1, Integrator5/1  "dz"
  Integrator5/1 -> z/1  "z"
  tau_phi/1 -> Integrator6/1  "ddphi"
  Integrator6/1 -> dphi/1, Integrator7/1  "dphi"
  Integrator7/1 -> Mux/1, phi/1  "phi"
  Integrator9/1 -> Mux/2, theta/1  "theta"
  Integrator8/1 -> dtheta/1, Integrator9/1  "dtheta"
  tau_theta/1 -> Integrator8/1  "ddtheta"
  Integrator11/1 -> Mux/3, psi/1  "psi"
  Integrator10/1 -> dpsi/1, Integrator11/1  "dpsi"
  tau_psi/1 -> Integrator10/1  "ddpsi"
  Mux/1 -> Demux/1  "(phi, theta, psi)"
  Demux/1 -> MATLAB Function3/2(phi), MATLAB Function4/2(phi), MATLAB Function/2(phi)
  Demux/2 -> MATLAB Function3/3(theta), MATLAB Function4/3(theta), MATLAB Function/3(theta)
  Demux/3 -> MATLAB Function/4(psi), MATLAB Function3/4(psi)

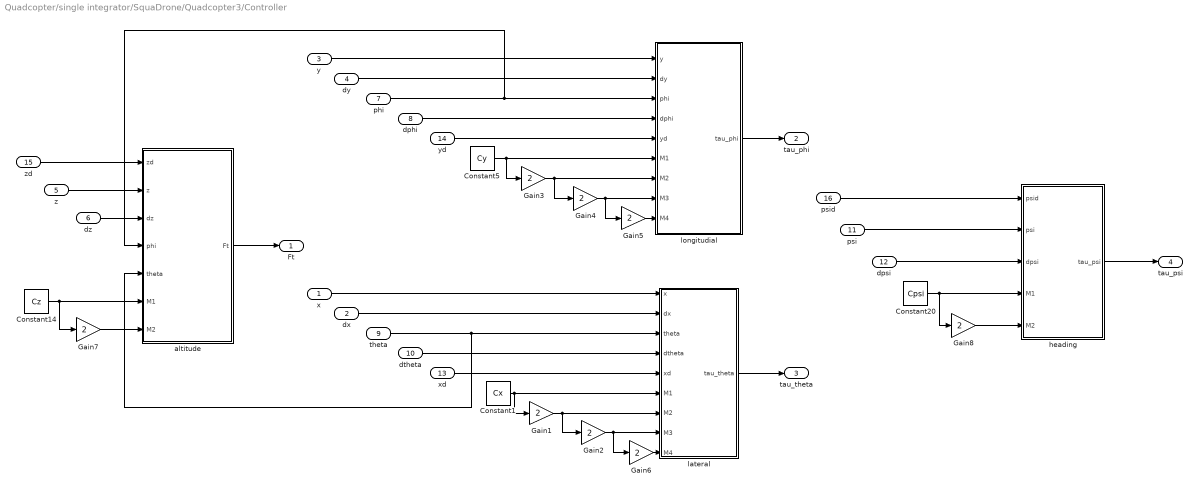
== system Quadcopter/single integrator/SquaDrone/Quadcopter3/Controller ==
  x : Inport
  dx : Inport  Port=2
  y : Inport  Port=3
  dy : Inport  Port=4
  z : Inport  Port=5
  dz : Inport  Port=6
  phi : Inport  Port=7
  dphi : Inport  Port=8
  theta : Inport  Port=9
  dtheta : Inport  Port=10
  psi : Inport  Port=11
  dpsi : Inport  Port=12
  xd : Inport  Port=13
  yd : Inport  Port=14
  zd : Inport  Port=15
  psid : Inport  Port=16
  Constant1 : Constant  Value=Cx
  Constant14 : Constant  Value=Cz
  Constant20 : Constant  Value=Cpsi
  Constant5 : Constant  Value=Cy
  Gain{1..8} (8 alike) : Gain  Gain=2
  altitude : MATLAB Function  TreatAsAtomicUnit=on
  heading : MATLAB Function  TreatAsAtomicUnit=on
  lateral : MATLAB Function  TreatAsAtomicUnit=on
  longitudial : MATLAB Function  TreatAsAtomicUnit=on
  Ft : Outport
  tau_phi : Outport  Port=2
  tau_theta : Outport  Port=3
  tau_psi : Outport  Port=4
  wires:
  altitude/1(Ft) -> Ft/1
  longitudial/1(tau_phi) -> tau_phi/1
  lateral/1(tau_theta) -> tau_theta/1
  heading/1(tau_psi) -> tau_psi/1
  Gain7/1 -> altitude/7(M2)
  Constant14/1 -> Gain7/1, altitude/6(M1)
  Constant20/1 -> Gain8/1, heading/4(M1)
  Gain8/1 -> heading/5(M2)
  psid/1 -> heading/1(psid)
  psi/1 -> heading/2(psi)
  dpsi/1 -> heading/3(dpsi)
  dx/1 -> lateral/2(dx)
  x/1 -> lateral/1(x)
  theta/1 -> lateral/3(theta), altitude/5(theta)
  dtheta/1 -> lateral/4(dtheta)
  y/1 -> longitudial/1(y)
  dy/1 -> longitudial/2(dy)
  phi/1 -> altitude/4(phi), longitudial/3(phi)
  dphi/1 -> longitudial/4(dphi)
  xd/1 -> lateral/5(xd)
  yd/1 -> longitudial/5(yd)
  zd/1 -> altitude/1(zd)
  z/1 -> altitude/2(z)
  dz/1 -> altitude/3(dz)
  Gain4/1 -> longitudial/8(M3), Gain5/1
  Constant5/1 -> longitudial/6(M1), Gain3/1
  Gain3/1 -> longitudial/7(M2), Gain4/1
  Gain5/1 -> longitudial/9(M4)
  Gain2/1 -> lateral/8(M3), Gain6/1
  Constant1/1 -> lateral/6(M1), Gain1/1
  Gain1/1 -> lateral/7(M2), Gain2/1
  Gain6/1 -> lateral/9(M4)

== system Quadcopter/single integrator/SquaDrone/Quadcopter3/Dynamic_System ==
  Ft : Inport
  tau_phi : Inport  Port=2
  tau_theta : Inport  Port=3
  tau_psi : Inport  Port=4
  Demux : Demux  Outputs=3
  Integrator{,1..11} (12 alike) : Integrator
  MATLAB Function : MATLAB Function  TreatAsAtomicUnit=on
  MATLAB Function3 : MATLAB Function  TreatAsAtomicUnit=on
  MATLAB Function4 : MATLAB Function  TreatAsAtomicUnit=on
  Mux : Mux  Inputs=3
  x : Outport
  dx : Outport  Port=2
  y : Outport  Port=3
  dy : Outport  Port=4
  z : Outport  Port=5
  dz : Outport  Port=6
  phi : Outport  Port=7
  dphi : Outport  Port=8
  theta : Outport  Port=9
  dtheta : Outport  Port=10
  psi : Outport  Port=11
  dpsi : Outport  Port=12
  wires:
  MATLAB Function3/1(ddx) -> Integrator/1  "ddx"
  Ft/1 -> MATLAB Function3/1(Ft), MATLAB Function4/1(Ft), MATLAB Function/1(Ft)
  Integrator/1 -> dx/1, Integrator1/1  "dx"
  Integrator1/1 -> x/1  "x"
  MATLAB Function/1(ddy) -> Integrator2/1  "ddy"
  Integrator2/1 -> dy/1, Integrator3/1  "dy"
  Integrator3/1 -> y/1  "y"
  MATLAB Function4/1(ddz) -> Integrator4/1  "ddz"
  Integrator4/1 -> dz/1, Integrator5/1  "dz"
  Integrator5/1 -> z/1  "z"
  tau_phi/1 -> Integrator6/1  "ddphi"
  Integrator6/1 -> dphi/1, Integrator7/1  "dphi"
  Integrator7/1 -> Mux/1, phi/1  "phi"
  Integrator9/1 -> Mux/2, theta/1  "theta"
  Integrator8/1 -> dtheta/1, Integrator9/1  "dtheta"
  tau_theta/1 -> Integrator8/1  "ddtheta"
  Integrator11/1 -> Mux/3, psi/1  "psi"
  Integrator10/1 -> dpsi/1, Integrator11/1  "dpsi"
  tau_psi/1 -> Integrator10/1  "ddpsi"
  Mux/1 -> Demux/1  "(phi, theta, psi)"
  Demux/1 -> MATLAB Function3/2(phi), MATLAB Function4/2(phi), MATLAB Function/2(phi)
  Demux/2 -> MATLAB Function3/3(theta), MATLAB Function4/3(theta), MATLAB Function/3(theta)
  Demux/3 -> MATLAB Function/4(psi), MATLAB Function3/4(psi)

== matlab function Quadcopter/single integrator/SquaDrone/Quadcopter2/Controller/altitude ==
  data: zd input; Ft output; z input; dz input; phi input; theta input; M1 input; M2 input
function Ft = fcn(zd, z, dz, phi, theta, M1, M2)
    
    Ft = (- allf.sat(dz + allf.sat(z - zd + dz, M1), M2) + 1) / (cos(phi) * cos(theta)); 
    
end

== matlab function Quadcopter/single integrator/SquaDrone/Quadcopter2/Controller/heading ==
  data: psid input; tau_psi output; psi input; dpsi input; M1 input; M2 input
function tau_psi = fcn(psid, psi, dpsi, M1, M2)

    tau_psi = - allf.sat(dpsi + allf.sat(psi - psid + dpsi, M1), M2);

end

== matlab function Quadcopter/single integrator/SquaDrone/Quadcopter2/Controller/lateral ==
  data: x input; dx input; theta input; dtheta input; xd input; M1 input; tau_theta output; M2 input; M3 input; M4 input
function tau_theta = fcn(x, dx, theta, dtheta, xd, M1, M2, M3, M4)
    
    z3 = dtheta + theta;
    z2 = dtheta + 2*theta - dx;
    z1 = dtheta + 3*theta - 3*dx - (x - xd);
    
    tau_theta = - allf.sat(dtheta + allf.sat(z3 + allf.sat(z2 + allf.sat(z1, M4), M3), M2), M1);

end

== matlab function Quadcopter/single integrator/SquaDrone/Quadcopter2/Controller/longitudial ==
  data: y input; dy input; phi input; dphi input; yd input; M1 input; tau_phi output; M2 input; M3 input; M4 input
function tau_phi = fcn(y, dy, phi, dphi, yd, M1, M2, M3, M4)

    z3 = dphi + phi;
    z2 = dphi + 2*phi + dy;
    z1 = dphi + 3*phi + 3*dy + y - yd;
    
    tau_phi =   - allf.sat(dphi + allf.sat(z3 + allf.sat(z2 + allf.sat(z1, M4), M3), M2), M1);

end

== matlab function Quadcopter/double integrator/SquaDrone/Drone1/Controller/altitude ==
  data: z input; dz input; phi input; theta input; zd input; Ft output; M1 input; M2 input
function Ft = fcn(z, dz, phi, theta, zd, M1, M2)
    
    Ft = (- allf.sat(dz + allf.sat(z - zd + dz, M1), M2) + 1) / (cos(phi) * cos(theta)); 
    
end

== matlab function Quadcopter/double integrator/SquaDrone/Drone1/Controller/heading ==
  data: psid input; tau_psi output; psi input; dpsi input; M1 input; M2 input
function tau_psi = fcn(psid, psi, dpsi, M1, M2)

    tau_psi = - allf.sat(dpsi + allf.sat(psi - psid + dpsi, M1), M2);

end

== matlab function Quadcopter/double integrator/SquaDrone/Drone1/Controller/lateral ==
  data: theta input; dtheta input; thetad input; dthetad input; M1 input; tau_theta output; M2 input
function tau_theta = fcn(theta, dtheta, thetad, dthetad, M1, M2)
    
    tau_theta = - allf.sat(dtheta - dthetad + allf.sat(theta - thetad + dtheta - dthetad, M1), M2);

end

== matlab function Quadcopter/double integrator/SquaDrone/Drone1/Controller/longitudial ==
  data: phi input; dphi input; phid input; dphid input; M1 input; tau_phi output; M2 input
function tau_phi = fcn(phi, dphi, phid, dphid, M1, M2)
    
    tau_phi = - allf.sat(dphi - dphid + allf.sat(phi - phid + dphi - dphid, M1), M2);

end

== matlab function Quadcopter/single integrator/SquaDrone/Quadcopter2/Dynamic_System/MATLAB Function ==
  data: Ft input; ddy output; phi input; theta input; psi input
function ddy = fcn(Ft, phi, theta, psi)
    
    ddy = Ft * cos(theta)*sin(phi);
    
end

== matlab function Quadcopter/single integrator/SquaDrone/Quadcopter2/Dynamic_System/MATLAB Function3 ==
  data: Ft input; ddx output; phi input; theta input; psi input
function ddx = fcn(Ft, phi, theta, psi)

    ddx = - Ft * sin(theta);
    
end

== matlab function Quadcopter/single integrator/SquaDrone/Quadcopter2/Dynamic_System/MATLAB Function4 ==
  data: Ft input; ddz output; phi input; theta input
function ddz = fcn(Ft, phi, theta)
    
    ddz = Ft * cos(theta)*cos(phi) - 1;
    
end

== matlab function Quadcopter/single integrator/SquaDrone/Quadcopter3/Controller/altitude ==
  data: zd input; Ft output; z input; dz input; phi input; theta input; M1 input; M2 input
function Ft = fcn(zd, z, dz, phi, theta, M1, M2)
    
    Ft = (- allf.sat(dz + allf.sat(z - zd + dz, M1), M2) + 1) / (cos(phi) * cos(theta)); 
    
end

== matlab function Quadcopter/single integrator/SquaDrone/Quadcopter3/Controller/heading ==
  data: psid input; tau_psi output; psi input; dpsi input; M1 input; M2 input
function tau_psi = fcn(psid, psi, dpsi, M1, M2)

    tau_psi = - allf.sat(dpsi + allf.sat(psi - psid + dpsi, M1), M2);

end

== matlab function Quadcopter/single integrator/SquaDrone/Quadcopter3/Controller/lateral ==
  data: x input; dx input; theta input; dtheta input; xd input; M1 input; tau_theta output; M2 input; M3 input; M4 input
function tau_theta = fcn(x, dx, theta, dtheta, xd, M1, M2, M3, M4)
    
    z3 = dtheta + theta;
    z2 = dtheta + 2*theta - dx;
    z1 = dtheta + 3*theta - 3*dx - (x - xd);
    
    tau_theta = - allf.sat(dtheta + allf.sat(z3 + allf.sat(z2 + allf.sat(z1, M4), M3), M2), M1);

end

== matlab function Quadcopter/single integrator/SquaDrone/Quadcopter3/Controller/longitudial ==
  data: y input; dy input; phi input; dphi input; yd input; M1 input; tau_phi output; M2 input; M3 input; M4 input
function tau_phi = fcn(y, dy, phi, dphi, yd, M1, M2, M3, M4)

    z3 = dphi + phi;
    z2 = dphi + 2*phi + dy;
    z1 = dphi + 3*phi + 3*dy + y - yd;
    
    tau_phi =   - allf.sat(dphi + allf.sat(z3 + allf.sat(z2 + allf.sat(z1, M4), M3), M2), M1);

end

== matlab function Quadcopter/single integrator/SquaDrone/Quadcopter3/Dynamic_System/MATLAB Function ==
  data: Ft input; ddy output; phi input; theta input; psi input
function ddy = fcn(Ft, phi, theta, psi)
    
    ddy = Ft * cos(theta)*sin(phi);
    
end

== matlab function Quadcopter/single integrator/SquaDrone/Quadcopter3/Dynamic_System/MATLAB Function3 ==
  data: Ft input; ddx output; phi input; theta input; psi input
function ddx = fcn(Ft, phi, theta, psi)

    ddx = - Ft * sin(theta);
    
end

== matlab function Quadcopter/single integrator/SquaDrone/Quadcopter3/Dynamic_System/MATLAB Function4 ==
  data: Ft input; ddz output; phi input; theta input
function ddz = fcn(Ft, phi, theta)
    
    ddz = Ft * cos(theta)*cos(phi) - 1;
    
end

== matlab function Quadcopter/double integrator/SquaDrone/Drone1/Dynamic_System/MATLAB Function ==
  data: Ft input; ddy output; phi input; theta input; psi input
function ddy = fcn(Ft, phi, theta, psi)
    
    ddy = Ft * cos(theta)*sin(phi);
    
end

== matlab function Quadcopter/double integrator/SquaDrone/Drone1/Dynamic_System/MATLAB Function3 ==
  data: Ft input; ddx output; phi input; theta input; psi input
function ddx = fcn(Ft, phi, theta, psi)

    ddx = - Ft * sin(theta);
    
end

== matlab function Quadcopter/double integrator/SquaDrone/Drone1/Dynamic_System/MATLAB Function4 ==
  data: Ft input; ddz output; phi input; theta input
function ddz = fcn(Ft, phi, theta)
    
    ddz = Ft * cos(theta)*cos(phi) - 1;
    
end

== matlab function Quadcopter/double integrator/SquaDrone/Drone2/Controller/altitude ==
  data: z input; dz input; phi input; theta input; zd input; Ft output; M1 input; M2 input
function Ft = fcn(z, dz, phi, theta, zd, M1, M2)
    
    Ft = (- allf.sat(dz + allf.sat(z - zd + dz, M1), M2) + 1) / (cos(phi) * cos(theta)); 
    
end

== matlab function Quadcopter/double integrator/SquaDrone/Drone2/Controller/heading ==
  data: psid input; tau_psi output; psi input; dpsi input; M1 input; M2 input
function tau_psi = fcn(psid, psi, dpsi, M1, M2)

    tau_psi = - allf.sat(dpsi + allf.sat(psi - psid + dpsi, M1), M2);

end

== matlab function Quadcopter/Quadcopter control xd, yd, zd, psid/Controller/altitude ==
  data: zd input; Ft output; z input; dz input; phi input; theta input; M1 input; M2 input
function Ft = fcn(zd, z, dz, phi, theta, M1, M2)
    
    Ft = (- allf.sat(dz + allf.sat(z - zd + dz, M1), M2) + 1) / (cos(phi) * cos(theta)); 
    
end

== matlab function Quadcopter/Quadcopter control xd, yd, zd, psid/Controller/longitudinal ==
  data: y input; dy input; phi input; dphi input; yd input; M1 input; tau_phi output; M2 input; M3 input; M4 input
function tau_phi = fcn(y, dy, phi, dphi, yd, M1, M2, M3, M4)

    z3 = dphi + phi;
    z2 = dphi + 2*phi + dy;
    z1 = dphi + 3*phi + 3*dy + y - yd;
    
    tau_phi =   - allf.sat(dphi + allf.sat(z3 + allf.sat(z2 + allf.sat(z1, M1), M2), M3), M4);

end

== matlab function Quadcopter/Quadcopter control xd, yd, zd, psid/Controller/heading ==
  data: psid input; tau_psi output; psi input; dpsi input; M1 input; M2 input
function tau_psi = fcn(psid, psi, dpsi, M1, M2)

    tau_psi = - allf.sat(dpsi + allf.sat(psi - psid + dpsi, M1), M2);

end

== matlab function Quadcopter/Quadcopter control xd, yd, zd, psid/Controller/lateral ==
  data: x input; dx input; theta input; dtheta input; xd input; M1 input; tau_theta output; M2 input; M3 input; M4 input
function tau_theta = fcn(x, dx, theta, dtheta, xd, M1, M2, M3, M4)
    
    z3 = dtheta + theta;
    z2 = dtheta + 2*theta - dx;
    z1 = dtheta + 3*theta - 3*dx - (x - xd);
    
    tau_theta = - allf.sat(dtheta + allf.sat(z3 + allf.sat(z2 + allf.sat(z1, M1), M2), M3), M4);
    
end

== matlab function Quadcopter/Quadcopter control xd, yd, zd, psid/Dynamic_System/MATLAB Function ==
  data: Ft input; ddy output; phi input; theta input; psi input
function ddy = fcn(Ft, phi, theta, psi)
    
    ddy = Ft * cos(theta)*sin(phi);
    
end

== matlab function Quadcopter/Quadcopter control xd, yd, zd, psid/Dynamic_System/MATLAB Function3 ==
  data: Ft input; ddx output; phi input; theta input; psi input
function ddx = fcn(Ft, phi, theta, psi)

    ddx = - Ft * sin(theta);
    
end

== matlab function Quadcopter/Quadcopter control xd, yd, zd, psid/Dynamic_System/MATLAB Function4 ==
  data: Ft input; ddz output; phi input; theta input
function ddz = fcn(Ft, phi, theta)
    
    ddz = Ft * cos(theta)*cos(phi) - 1;
    
end

== matlab function Quadcopter/double integrator/SquaDrone/Drone2/Controller/lateral ==
  data: theta input; dtheta input; thetad input; dthetad input; M1 input; tau_theta output; M2 input
function tau_theta = fcn(theta, dtheta, thetad, dthetad, M1, M2)
    
    tau_theta = - allf.sat(dtheta - dthetad + allf.sat(theta - thetad + dtheta - dthetad, M1), M2);

end

== matlab function Quadcopter/double integrator/SquaDrone/Drone2/Controller/longitudial ==
  data: phi input; dphi input; phid input; dphid input; M1 input; tau_phi output; M2 input
function tau_phi = fcn(phi, dphi, phid, dphid, M1, M2)
    
    tau_phi = - allf.sat(dphi - dphid + allf.sat(phi - phid + dphi - dphid, M1), M2);

end

== matlab function Quadcopter/double integrator/SquaDrone/Drone2/Dynamic_System/MATLAB Function ==
  data: Ft input; ddy output; phi input; theta input; psi input
function ddy = fcn(Ft, phi, theta, psi)
    
    ddy = Ft * cos(theta)*sin(phi);
    
end

== matlab function Quadcopter/double integrator/SquaDrone/Drone2/Dynamic_System/MATLAB Function3 ==
  data: Ft input; ddx output; phi input; theta input; psi input
function ddx = fcn(Ft, phi, theta, psi)

    ddx = - Ft * sin(theta);
    
end

== matlab function Quadcopter/double integrator/SquaDrone/Drone2/Dynamic_System/MATLAB Function4 ==
  data: Ft input; ddz output; phi input; theta input
function ddz = fcn(Ft, phi, theta)
    
    ddz = Ft * cos(theta)*cos(phi) - 1;
    
end

== matlab function Quadcopter/double integrator/SquaDrone/Drone3/Controller/altitude ==
  data: z input; dz input; phi input; theta input; zd input; Ft output; M1 input; M2 input
function Ft = fcn(z, dz, phi, theta, zd, M1, M2)
    
    Ft = (- allf.sat(dz + allf.sat(z - zd + dz, M1), M2) + 1) / (cos(phi) * cos(theta)); 
    
end

== matlab function Quadcopter/double integrator/SquaDrone/Drone3/Controller/heading ==
  data: psid input; tau_psi output; psi input; dpsi input; M1 input; M2 input
function tau_psi = fcn(psid, psi, dpsi, M1, M2)

    tau_psi = - allf.sat(dpsi + allf.sat(psi - psid + dpsi, M1), M2);

end

== matlab function Quadcopter/double integrator/SquaDrone/Drone3/Controller/lateral ==
  data: theta input; dtheta input; thetad input; dthetad input; M1 input; tau_theta output; M2 input
function tau_theta = fcn(theta, dtheta, thetad, dthetad, M1, M2)
    
    tau_theta = - allf.sat(dtheta - dthetad + allf.sat(theta - thetad + dtheta - dthetad, M1), M2);

end

== matlab function Quadcopter/double integrator/SquaDrone/Drone3/Controller/longitudial ==
  data: phi input; dphi input; phid input; dphid input; M1 input; tau_phi output; M2 input
function tau_phi = fcn(phi, dphi, phid, dphid, M1, M2)
    
    tau_phi = - allf.sat(dphi - dphid + allf.sat(phi - phid + dphi - dphid, M1), M2);

end

== matlab function Quadcopter/double integrator/SquaDrone/Drone3/Dynamic_System/MATLAB Function ==
  data: Ft input; ddy output; phi input; theta input; psi input
function ddy = fcn(Ft, phi, theta, psi)
    
    ddy = Ft * cos(theta)*sin(phi);
    
end

== matlab function Quadcopter/double integrator/SquaDrone/Drone3/Dynamic_System/MATLAB Function3 ==
  data: Ft input; ddx output; phi input; theta input; psi input
function ddx = fcn(Ft, phi, theta, psi)

    ddx = - Ft * sin(theta);
    
end

== matlab function Quadcopter/double integrator/SquaDrone/Drone3/Dynamic_System/MATLAB Function4 ==
  data: Ft input; ddz output; phi input; theta input
function ddz = fcn(Ft, phi, theta)
    
    ddz = Ft * cos(theta)*cos(phi) - 1;
    
end

== matlab function Quadcopter/scheme - simple system_double integrator/Path Tracking Controller  ==
  data: x1 input; dx1 input; u1 output; x2 input; dx2 input; x3 input; dx3 input; x_cmd input; dx_cmd input; k input; b1 input; b2 input; b3 input; u2 output; u3 output; r_12 input; r_32 input
function [u1, u2, u3] = fcn(x1, dx1, x2, dx2, x3, dx3, x_cmd, dx_cmd, k, b1, b2, b3, r_12, r_32)
    
    u1 = - (1 + k) * dx1 - k * x1 + dx2 + k * x2 - b1 * dx3 - b1 * k * x3 + b1 * (k + 1) * dx_cmd + b1 * k * x_cmd + k * r_12;

    u2 = b2 * u1 + (b2 * k + 1) * dx1 + k * x1 - (k + 2) * dx2 - 2 * k * x2 + dx3 + k * x3 - k * r_x12 - k * r_32;
    
    u3 = b3 * u2 + (b3*k + 1)*dx2 + k * x2 - (k + 1)*dx3 - k*x3 + k * r_32;
    
end

== matlab function Quadcopter/scheme - double integrator/SquaDrone/Drone1/Controller/altitude ==
  data: z input; dz input; phi input; theta input; zd input; Ft output; M1 input; M2 input
function Ft = fcn(z, dz, phi, theta, zd, M1, M2)
    
    Ft = (- allf.sat(dz + allf.sat(z - zd + dz, M1), M2) + 1) / (cos(phi) * cos(theta)); 
    
end

== matlab function Quadcopter/scheme - double integrator/SquaDrone/Drone1/Controller/heading ==
  data: psid input; tau_psi output; psi input; dpsi input; M1 input; M2 input
function tau_psi = fcn(psid, psi, dpsi, M1, M2)

    tau_psi = - allf.sat(dpsi + allf.sat(psi - psid + dpsi, M1), M2);

end

== matlab function Quadcopter/scheme - double integrator/SquaDrone/Drone1/Controller/lateral ==
  data: theta input; dtheta input; thetad input; dthetad input; M1 input; tau_theta output; M2 input
function tau_theta = fcn(theta, dtheta, thetad, dthetad, M1, M2)
    
    tau_theta = - allf.sat(dtheta + allf.sat(theta - thetad + dtheta - dthetad, M1), M2);

end

== matlab function Quadcopter/scheme - double integrator/SquaDrone/Drone1/Controller/longitudial ==
  data: phi input; dphi input; phid input; dphid input; M1 input; tau_phi output; M2 input
function tau_phi = fcn(phi, dphi, phid, dphid, M1, M2)
    
    tau_phi = - allf.sat(dphi + allf.sat(phi - phid + dphi - dphid, M1), M2);

end

== matlab function Quadcopter/scheme - double integrator/SquaDrone/Drone1/Dynamic_System/MATLAB Function ==
  data: Ft input; ddy output; phi input; theta input; psi input
function ddy = fcn(Ft, phi, theta, psi)
    
    ddy = Ft * cos(theta)*sin(phi);
    
end

== matlab function Quadcopter/scheme - double integrator/SquaDrone/Drone1/Dynamic_System/MATLAB Function3 ==
  data: Ft input; ddx output; phi input; theta input; psi input
function ddx = fcn(Ft, phi, theta, psi)

    ddx = - Ft * sin(theta);
    
end

== matlab function Quadcopter/scheme - double integrator/SquaDrone/Drone1/Dynamic_System/MATLAB Function4 ==
  data: Ft input; ddz output; phi input; theta input
function ddz = fcn(Ft, phi, theta)
    
    ddz = Ft * cos(theta)*cos(phi) - 1;
    
end
